simulink model "Exercise5"  (R2019b)
settings: Solver=VariableStepAuto  StartTime=0.0  StopTime=10.0  RelTol=1e-3
libraries: fuzblock x1
settings Model: Creator=victo  LastModifiedBy=victo
settings OptimizationCC: BooleanDataType=off

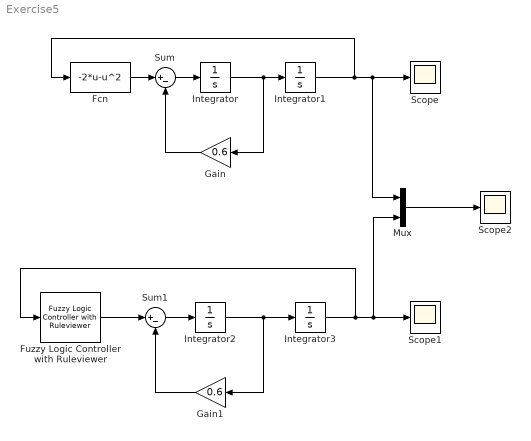
== system Exercise5 ==
  Fcn : Fcn  Expr=-2*u-u^2
  Fuzzy Logic Controller with Ruleviewer : fuzblock/Fuzzy Logic  Controller  with Ruleviewer  fismatrix=fismat1  Ts=2
  Gain : Gain  Gain=0.6
  Gain1 : Gain  Gain=0.6
  Integrator : Integrator  InitialCondition=0.5
  Integrator1 : Integrator  InitialCondition=-0.2
  Integrator2 : Integrator  InitialCondition=0.5
  Integrator3 : Integrator  InitialCondition=-0.2
  Mux : Mux  Inputs=2
  Scope : Scope
  Scope1 : Scope
  Scope2 : Scope
  Sum : Sum  Inputs=|+-
  Sum1 : Sum  Inputs=|+-
  wires:
  Sum/1 -> Integrator/1
  Integrator/1 -> Integrator1/1, Gain/1
  Gain/1 -> Sum/2
  Fcn/1 -> Sum/1
  Integrator1/1 -> Fcn/1, Mux/1, Scope/1
  Gain1/1 -> Sum1/2
  Integrator3/1 -> Mux/2, Scope1/1, Fuzzy Logic Controller with Ruleviewer/1
  Integrator2/1 -> Integrator3/1, Gain1/1
  Fuzzy Logic Controller with Ruleviewer/1 -> Sum1/1
  Sum1/1 -> Integrator2/1
  Mux/1 -> Scope2/1
